simulink model "softSwitch"  (R2018b)
settings: Solver=FixedStepAuto  StartTime=0.0  StopTime=50  FixedStep=0.01  RelTol=1e-3
undefined symbols (not defined in the file): DiscIntNeverNeededParam
settings Model: Creator=wout7  LastModifiedBy=wout7

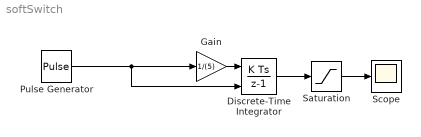
== system softSwitch ==
  Discrete-Time Integrator : DiscreteIntegrator  ExternalReset=either  SampleTime=-1  ICPrevOutput=DiscIntNeverNeededParam  ICPrevScaledInput=DiscIntNeverNeededParam
  Gain : Gain  Gain=1/(5)
  Pulse Generator : DiscretePulseGenerator  PulseType=Time based  Period=11  PulseWidth=50
  Saturation : Saturate  UpperLimit=1  LowerLimit=0
  Scope : Scope
  wires:
  Gain/1 -> Discrete-Time Integrator/1
  Discrete-Time Integrator/1 -> Saturation/1
  Saturation/1 -> Scope/1
  Pulse Generator/1 -> Discrete-Time Integrator/2, Gain/1
